simulink model "dronesmodel_wofb"  (R2015b)
settings: Solver=VariableStepAuto  StartTime=0.0  StopTime=100  RelTol=1e-3
values from neighbouring files (symbols this model uses):
  De = 7.7*10^(-6)    (= 7.7e-06)    [mainDrones.m]
  Je = 3*10^(-6)    (= 3e-06)    [mainDrones.m]
  Kb = 0.171    [mainDrones.m]
  Kt = 0.171    [mainDrones.m]
  La = 14.8*10^(-3)    (= 0.0148)    [mainDrones.m]
  Ra = 25.6    [mainDrones.m]
libraries: simulink x2
settings Model: Creator=Kelvin  LastModifiedBy=Kelvin

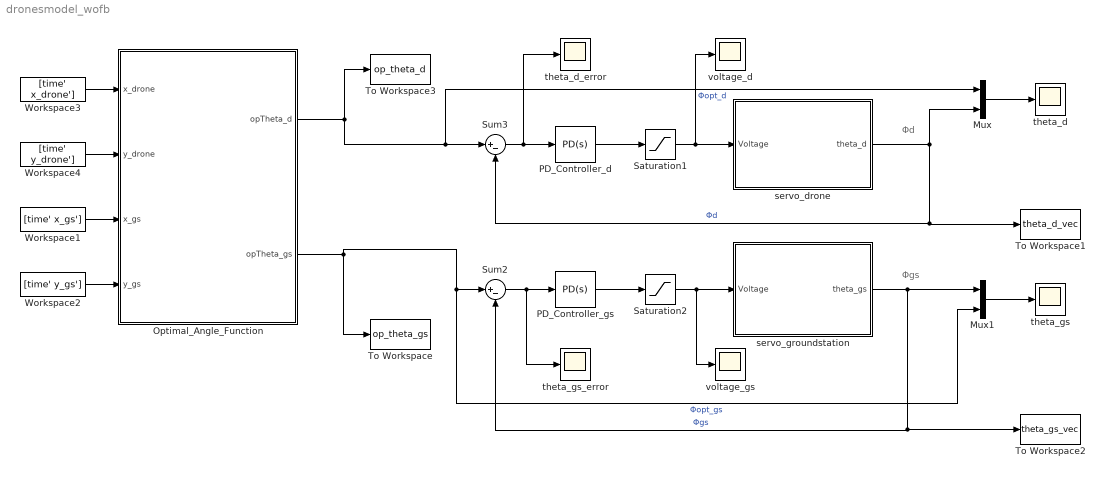
== system dronesmodel_wofb ==
  note: Φgs
  note: Φd
  Mux : Mux  Inputs=2
  Mux1 : Mux  Inputs=2
  "Optimal_Angle_Function " : MATLAB Function  TreatAsAtomicUnit=on
  PD_Controller_d : simulink/Continuous/PID Controller  Controller=PD  TimeDomain=Continuous-time  SampleTime=-1  IntegratorMethod=Forward Euler  FilterMethod=Forward Euler  Form=Parallel  UseFilter=on  ControllerParametersSource=internal  P=739.414726834109  I=0.0172882676140403  D=150.790271020884  N=52.8940738192282  InitialConditionSource=internal  InitialConditionForIntegrator=0  InitialConditionForFilter=0  ExternalReset=none  LimitOutput=off  UpperSaturationLimit=inf  LowerSaturationLimit=-inf  LinearizeAsGain=on  AntiWindupMode=none  Kb=1  TrackingMode=off  Kt=1  PParamMin=[]  PParamMax=[]  IParamMin=[]  IParamMax=[]  DParamMin=[]  DParamMax=[]  NParamMin=[]  NParamMax=[]  KbParamMin=[]  KbParamMax=[]  KtParamMin=[]  KtParamMax=[]  POutMin=[]  POutMax=[]  IOutMin=[]  IOutMax=[]  DOutMin=[]  DOutMax=[]  NOutMin=[]  NOutMax=[]  KbOutMin=[]  KbOutMax=[]  KtOutMin=[]  KtOutMax=[]  IntegratorOutMin=[]  IntegratorOutMax=[]  FilterOutMin=[]  FilterOutMax=[]  SumOutMin=[]  SumOutMax=[]  SumI1OutMin=[]  SumI1OutMax=[]  SumI2OutMin=[]  SumI2OutMax=[]  SumI3OutMin=[]  SumI3OutMax=[]  SumDOutMin=[]  SumDOutMax=[]  SaturationOutMin=[]  SaturationOutMax=[]  IntegratorContinuousStateAttributes=''  IntegratorStateMustResolveToSignalObject=off  IntegratorRTWStateStorageClass=Auto  FilterContinuousStateAttributes=''  FilterStateMustResolveToSignalObject=off  FilterRTWStateStorageClass=Auto  DifferentiatorICPrevScaledInput=0  DifferentiatorOutMin=[]  DifferentiatorOutMax=[]
  PD_Controller_gs : simulink/Continuous/PID Controller  Controller=PD  TimeDomain=Continuous-time  SampleTime=-1  IntegratorMethod=Forward Euler  FilterMethod=Forward Euler  Form=Parallel  UseFilter=on  ControllerParametersSource=internal  P=739.414726834109  I=0.0172882676140403  D=150.790271020884  N=52.8940738192282  InitialConditionSource=internal  InitialConditionForIntegrator=0  InitialConditionForFilter=0  ExternalReset=none  LimitOutput=off  UpperSaturationLimit=inf  LowerSaturationLimit=-inf  LinearizeAsGain=on  AntiWindupMode=none  Kb=1  TrackingMode=off  Kt=1  PParamMin=[]  PParamMax=[]  IParamMin=[]  IParamMax=[]  DParamMin=[]  DParamMax=[]  NParamMin=[]  NParamMax=[]  KbParamMin=[]  KbParamMax=[]  KtParamMin=[]  KtParamMax=[]  POutMin=[]  POutMax=[]  IOutMin=[]  IOutMax=[]  DOutMin=[]  DOutMax=[]  NOutMin=[]  NOutMax=[]  KbOutMin=[]  KbOutMax=[]  KtOutMin=[]  KtOutMax=[]  IntegratorOutMin=[]  IntegratorOutMax=[]  FilterOutMin=[]  FilterOutMax=[]  SumOutMin=[]  SumOutMax=[]  SumI1OutMin=[]  SumI1OutMax=[]  SumI2OutMin=[]  SumI2OutMax=[]  SumI3OutMin=[]  SumI3OutMax=[]  SumDOutMin=[]  SumDOutMax=[]  SaturationOutMin=[]  SaturationOutMax=[]  IntegratorContinuousStateAttributes=''  IntegratorStateMustResolveToSignalObject=off  IntegratorRTWStateStorageClass=Auto  FilterContinuousStateAttributes=''  FilterStateMustResolveToSignalObject=off  FilterRTWStateStorageClass=Auto  DifferentiatorICPrevScaledInput=0  DifferentiatorOutMin=[]  DifferentiatorOutMax=[]
  Saturation1 : Saturate  UpperLimit=10  LowerLimit=-10
  Saturation2 : Saturate  UpperLimit=10  LowerLimit=-10
  Sum2 : Sum  Inputs=|+-
  Sum3 : Sum  Inputs=|+-
  To Workspace : ToWorkspace  VariableName=op_theta_gs  SaveFormat=Timeseries  SampleTime=-1
  To Workspace1 : ToWorkspace  VariableName=theta_d_vec  SaveFormat=Timeseries  SampleTime=-1
  To Workspace2 : ToWorkspace  VariableName=theta_gs_vec  SaveFormat=Timeseries  SampleTime=-1
  To Workspace3 : ToWorkspace  VariableName=op_theta_d  SaveFormat=Timeseries  SampleTime=-1
  Workspace1 : FromWorkspace  VariableName=[time' x_gs']  SampleTime=1
  Workspace2 : FromWorkspace  VariableName=[time' y_gs']  SampleTime=1
  Workspace3 : FromWorkspace  VariableName=[time' x_drone']  SampleTime=1
  Workspace4 : FromWorkspace  VariableName=[time' y_drone']  OutDataTypeStr=double  SampleTime=1
  servo_drone : Subsystem
  servo_groundstation : Subsystem
  theta_d : Scope
  theta_d_error : Scope
  theta_gs : Scope
  theta_gs_error : Scope
  voltage_d : Scope
  voltage_gs : Scope
  wires:
  "Optimal_Angle_Function "/2(opTheta_gs) -> Mux1/2, Sum2/1, To Workspace/1  "Φopt_gs"
  PD_Controller_d/1 -> Saturation1/1
  PD_Controller_gs/1 -> Saturation2/1
  Saturation2/1 -> voltage_gs/1, servo_groundstation/1(Voltage)
  Saturation1/1 -> voltage_d/1, servo_drone/1(Voltage)
  servo_drone/1(theta_d) -> To Workspace1/1, Sum3/2, Mux/2  "Φd"
  servo_groundstation/1(theta_gs) -> Sum2/2, To Workspace2/1, Mux1/1  "Φgs"
  Sum3/1 -> theta_d_error/1, PD_Controller_d/1
  "Optimal_Angle_Function "/1(opTheta_d) -> To Workspace3/1, Mux/1, Sum3/1  "Φopt_d"
  Sum2/1 -> theta_gs_error/1, PD_Controller_gs/1
  Mux/1 -> theta_d/1
  Mux1/1 -> theta_gs/1
  Workspace1/1 -> "Optimal_Angle_Function "/3(x_gs)
  Workspace2/1 -> "Optimal_Angle_Function "/4(y_gs)
  Workspace4/1 -> "Optimal_Angle_Function "/2(y_drone)
  Workspace3/1 -> "Optimal_Angle_Function "/1(x_drone)

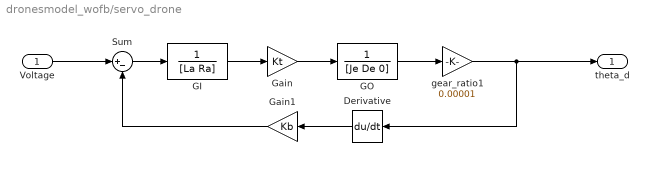
== system dronesmodel_wofb/servo_drone ==
  Voltage : Inport
  Derivative : Derivative
  GI : TransferFcn  Denominator=[La Ra]
  GO : TransferFcn  Denominator=[Je De 0]
  Gain : Gain  Gain=Kt
  Gain1 : Gain  Gain=Kb
  Sum : Sum  Inputs=|+-
  "gear_ratio1 " : Gain  Gain=0.00001
  theta_d : Outport
  wires:
  GO/1 -> "gear_ratio1 "/1
  Derivative/1 -> Gain1/1
  Sum/1 -> GI/1
  GI/1 -> Gain/1
  Gain1/1 -> Sum/2
  Gain/1 -> GO/1
  "gear_ratio1 "/1 -> theta_d/1, Derivative/1
  Voltage/1 -> Sum/1

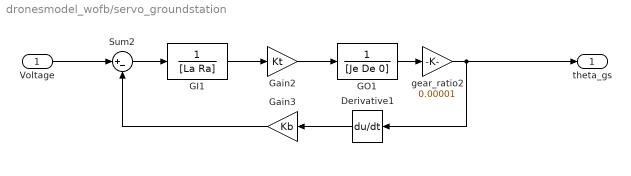
== system dronesmodel_wofb/servo_groundstation ==
  Voltage : Inport
  Derivative1 : Derivative
  GI1 : TransferFcn  Denominator=[La Ra]
  GO1 : TransferFcn  Denominator=[Je De 0]
  Gain2 : Gain  Gain=Kt
  Gain3 : Gain  Gain=Kb
  Sum2 : Sum  Inputs=|+-
  gear_ratio2 : Gain  Gain=0.00001
  theta_gs : Outport
  wires:
  GI1/1 -> Gain2/1
  Gain2/1 -> GO1/1
  Derivative1/1 -> Gain3/1
  Gain3/1 -> Sum2/2
  Sum2/1 -> GI1/1
  Voltage/1 -> Sum2/1
  gear_ratio2/1 -> theta_gs/1, Derivative1/1
  GO1/1 -> gear_ratio2/1

== matlab function dronesmodel_wofb/Optimal_Angle_Function  ==
  data: x_drone input; y_drone input; x_gs input; y_gs input; opTheta_d output; opTheta_gs output
function [opTheta_d,opTheta_gs] = system_2D_sim(x_drone,y_drone,x_gs,y_gs)
% put here the description of the function
% put here the description of the function
% put here the description of the function
% put here the description of the function

    % Optimal angles
    if y_drone > y_gs
        opt_theta_gs = atan2(y_drone-y_gs,x_drone-x_gs);
        opt_theta_d = pi + opt_theta_gs;
    else
        opt_theta_d = atan2(y_gs-y_drone,x_gs-x_drone);
        opt_theta_gs = pi + opt_theta_d;
    end
    
    % (OUTPUT) Optimal angles for groundstation and drone 
    opTheta_gs = atan2(y_drone-y_gs,x_drone-x_gs);
    opTheta_d  = opTheta_gs - pi;
 
end
